simulink model "Rocket_Simulation"  (R2024a)
settings: Solver=VariableStepAuto  StartTime=0.0  StopTime=30  RelTol=1e-3
values from neighbouring files (symbols this model uses):
  g = -9.80665    [OpenRocketDataLoader.m]
libraries: simulink x1, aerolibactuator x1, aerolibatmos2 x1
settings Model: Creator=bennettbabu  LastModifiedBy=bennettbabu

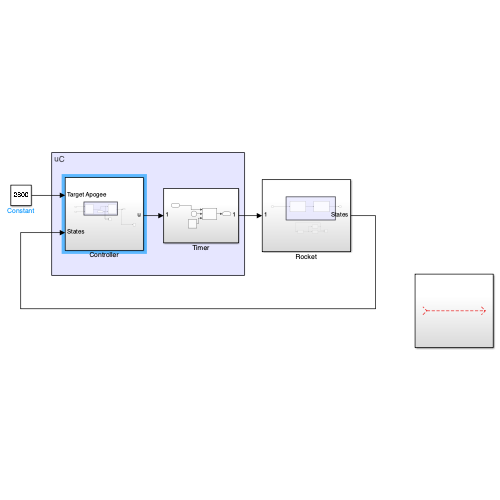
[thumbnail: Simulink's stored preview of the top-level diagram]
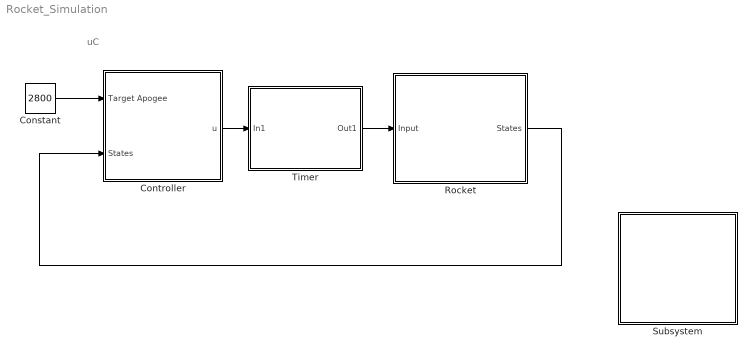
== system Rocket_Simulation ==
  note: uC
  Constant : Constant  Value=2800
  Controller : Subsystem
  Rocket : Subsystem
  Subsystem : Subsystem
  Timer : Subsystem
  wires:
  Rocket/1(States) -> Controller/2(States)
  Constant/1 -> Controller/1(Target Apogee)
  Controller/1(u) -> Timer/1(In1)
  Timer/1(Out1) -> Rocket/1(Input)

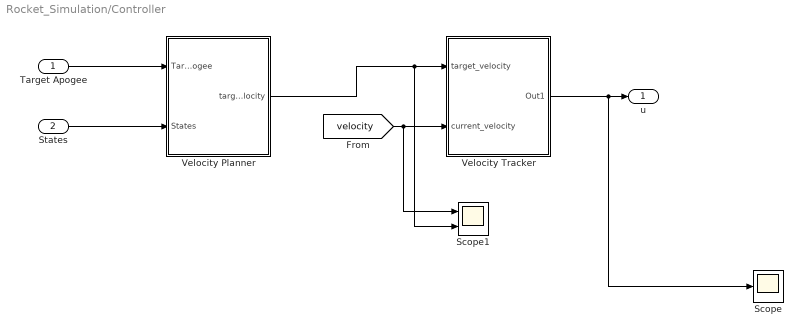
== system Rocket_Simulation/Controller ==
  Target Apogee : Inport
  States : Inport  Port=2
  Scope : Scope
  Scope1 : Scope  NumInputPorts=2
  Velocity Planner : Subsystem
  Velocity Tracker : Subsystem
  u : Outport
  wires:
  Target Apogee/1 -> Velocity Planner/1(Target Apogee)
  States/1 -> Velocity Planner/2(States)
  Velocity Tracker/1(Out1) -> Scope/1, u/1
  [velocity] -> Scope1/1, Velocity Tracker/2(current_velocity)
  Velocity Planner/1(target_velocity) -> Scope1/2, Velocity Tracker/1(target_velocity)

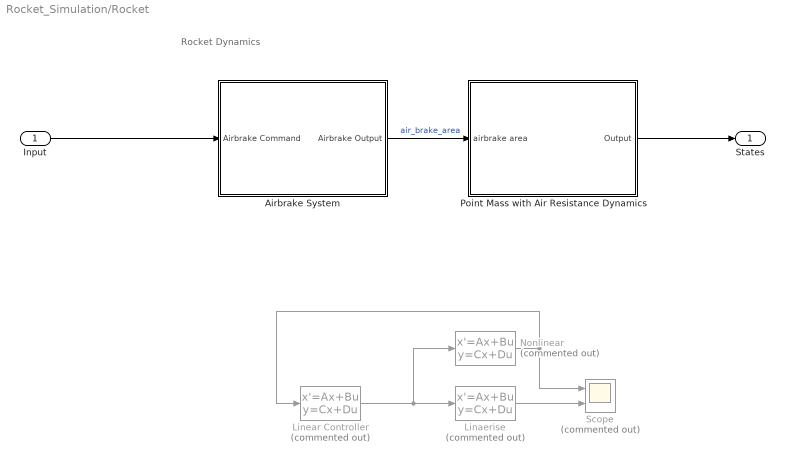
== system Rocket_Simulation/Rocket ==
  note: Rocket Dynamics
  Input : Inport
  Airbrake System : Subsystem
      mask Display: image('airbrake.png');
  "Linaerise " : StateSpace  Commented=on  InitialCondition=0
  Linear Controller : StateSpace  Commented=on  InitialCondition=0
  Nonlinear : StateSpace  Commented=on  InitialCondition=0
  "Point Mass with Air Resistance Dynamics " : Subsystem
      mask Display: image('rocket.jpeg');
  Scope : Scope  Commented=on  NumInputPorts=2
  States : Outport
  wires:
  "Point Mass with Air Resistance Dynamics "/1(Output) -> States/1
  Linear Controller/1 -> Nonlinear/1, "Linaerise "/1
  Nonlinear/1 -> Linear Controller/1, Scope/1
  "Linaerise "/1 -> Scope/2
  Input/1 -> Airbrake System/1(Airbrake Command)
  Airbrake System/1(Airbrake Output) -> "Point Mass with Air Resistance Dynamics "/1(airbrake area)  "air_brake_area"

== system Rocket_Simulation/Subsystem ==
  wires:
  ? -> ?

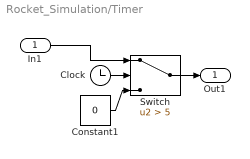
== system Rocket_Simulation/Timer ==
  In1 : Inport
  Clock : Clock
  Constant1 : Constant  Value=0
  Switch : Switch  Criteria=u2 > Threshold  Threshold=5  SaturateOnIntegerOverflow=off  InputSameDT=off
  Out1 : Outport
  wires:
  Switch/1 -> Out1/1
  Clock/1 -> Switch/2
  In1/1 -> Switch/1
  Constant1/1 -> Switch/3

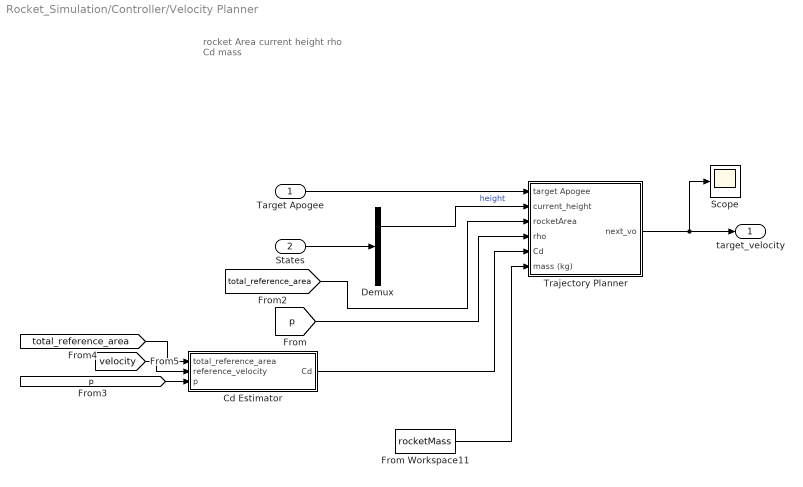
== system Rocket_Simulation/Controller/Velocity Planner ==
  note: rocket Area
      | current height
      | rho
      | Cd
      | mass
  Target Apogee : Inport
  States : Inport  Port=2
  Cd Estimator : Subsystem
  Demux : Demux  Outputs=2
  From Workspace11 : FromWorkspace  VariableName=rocketMass
  Scope : Scope
  Trajectory Planner : Subsystem
  target_velocity : Outport
  wires:
  States/1 -> Demux/1
  Demux/1 -> Trajectory Planner/2(current_height)  "height"
  Target Apogee/1 -> Trajectory Planner/1(target Apogee)
  [p] -> Trajectory Planner/4(rho)
  From Workspace11/1 -> Trajectory Planner/6(mass (kg))
  [p] -> Cd Estimator/3(p)
  [velocity] -> Cd Estimator/2(reference_velocity)
  [total_reference_area] -> Cd Estimator/1(total_reference_area)
  [total_reference_area] -> Trajectory Planner/3(rocketArea)
  Trajectory Planner/1(next_vo) -> Scope/1, target_velocity/1
  Cd Estimator/1(Cd) -> Trajectory Planner/5(Cd)

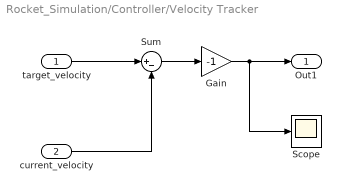
== system Rocket_Simulation/Controller/Velocity Tracker ==
  target_velocity : Inport
  current_velocity : Inport  Port=2
  Gain : Gain  Gain=-1
  Scope : Scope
  Sum : Sum  Inputs=|+-
  Out1 : Outport
  wires:
  Gain/1 -> Scope/1, Out1/1
  target_velocity/1 -> Sum/1
  current_velocity/1 -> Sum/2
  Sum/1 -> Gain/1

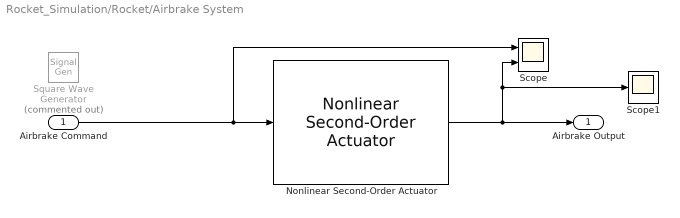
== system Rocket_Simulation/Rocket/Airbrake System ==
  Airbrake Command : Inport
  Nonlinear Second-Order Actuator : aerolibactuator/Nonlinear Second-Order Actuator  wn_fin=10  z_fin=0.7  fin_max=maxAirbrakeArea  fin_min=0  fin_maxrate=0.4  fin_act_0=0  fin_act_vel=0
  Scope : Scope  NumInputPorts=2
  Scope1 : Scope
  Square Wave Generator : SignalGenerator  Commented=on  WaveForm=square  Amplitude=0.01  Units=rad/sec
  Airbrake Output : Outport
  wires:
  Nonlinear Second-Order Actuator/1 -> Scope1/1, Scope/2, Airbrake Output/1
  Airbrake Command/1 -> Nonlinear Second-Order Actuator/1, Scope/1

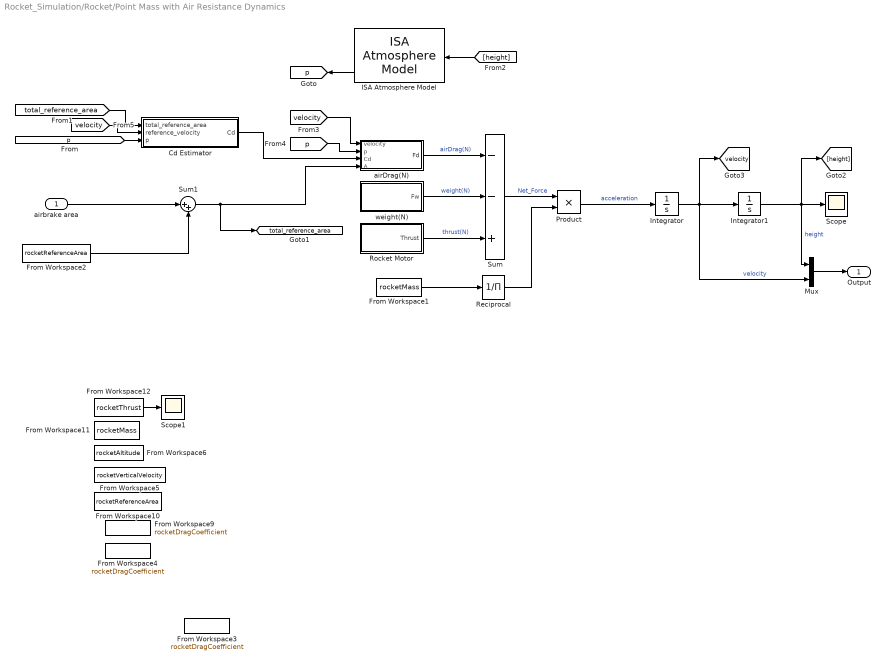
== system Rocket_Simulation/Rocket/Point Mass with Air Resistance Dynamics  ==
  airbrake area : Inport
  Cd Estimator : Subsystem
  From Workspace1 : FromWorkspace  VariableName=rocketMass
  From Workspace10 : FromWorkspace  VariableName=rocketReferenceArea
  From Workspace11 : FromWorkspace  VariableName=rocketMass
  From Workspace12 : FromWorkspace  VariableName=rocketThrust
  From Workspace2 : FromWorkspace  VariableName=rocketReferenceArea
  From Workspace3 : FromWorkspace  VariableName=rocketDragCoefficient
  From Workspace4 : FromWorkspace  VariableName=rocketDragCoefficient
  From Workspace5 : FromWorkspace  VariableName=rocketVerticalVelocity
  From Workspace6 : FromWorkspace  VariableName=rocketAltitude
  From Workspace9 : FromWorkspace  VariableName=rocketDragCoefficient
  ISA Atmosphere Model : aerolibatmos2/ISA Atmosphere Model  useExtended=off  action=Warning  custom=off  viscosityOut=off  g=9.80665  gamma=1.4  R=287.0531  L=0.0065  h_trop=11000  h_strat=20000  rho0=1.225  P0=101325  T0=288.15  h0=0  S=110.4  Tref=273.15  muref=1.716e-5
  Integrator : Integrator
  Integrator1 : Integrator
  Mux : Mux  Inputs=2
  Product : Product
  Reciprocal : Product  Inputs=/
  "Rocket Motor " : Subsystem
  Scope : Scope
  Scope1 : Scope
  Sum : Sum  Inputs=--+
  Sum1 : Sum  Inputs=|++
  airDrag(N) : Subsystem
  weight(N) : Subsystem
  Output : Outport
  tag scope: p=global, total_reference_area=global, velocity=global
  wires:
  "Rocket Motor "/1(Thrust) -> Sum/3  "thrust(N)"
  airDrag(N)/1(Fd) -> Sum/1  "airDrag(N)"
  weight(N)/1(Fw) -> Sum/2  "weight(N)"
  Sum/1 -> Product/1  "Net_Force"
  [p] -> Cd Estimator/3(p)
  ISA Atmosphere Model/4 -> [p]
  [total_reference_area] -> Cd Estimator/1(total_reference_area)
  [height] -> ISA Atmosphere Model/1
  [velocity] -> airDrag(N)/1(velocity)
  [p] -> airDrag(N)/2(p)
  Product/1 -> Integrator/1  "acceleration"
  Integrator/1 -> [velocity], Integrator1/1, Mux/2  "velocity"
  Integrator1/1 -> Mux/1, [height], Scope/1  "height"
  Mux/1 -> Output/1
  [velocity] -> Cd Estimator/2(reference_velocity)
  Reciprocal/1 -> Product/2
  From Workspace1/1 -> Reciprocal/1
  From Workspace12/1 -> Scope1/1
  airbrake area/1 -> Sum1/1
  Sum1/1 -> [total_reference_area], airDrag(N)/4(A)
  From Workspace2/1 -> Sum1/2
  Cd Estimator/1(Cd) -> airDrag(N)/3(Cd)

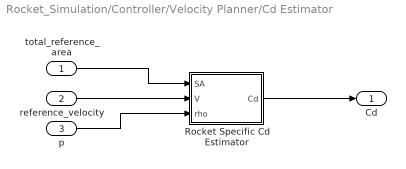
== system Rocket_Simulation/Controller/Velocity Planner/Cd Estimator ==
  total_reference_area : Inport
  reference_velocity : Inport  Port=2
  p : Inport  Port=3
  Rocket Specific Cd Estimator : MATLAB Function  TreatAsAtomicUnit=on
  Cd : Outport
  wires:
  Rocket Specific Cd Estimator/1(Cd) -> Cd/1
  total_reference_area/1 -> Rocket Specific Cd Estimator/1(SA)
  reference_velocity/1 -> Rocket Specific Cd Estimator/2(V)
  p/1 -> Rocket Specific Cd Estimator/3(rho)

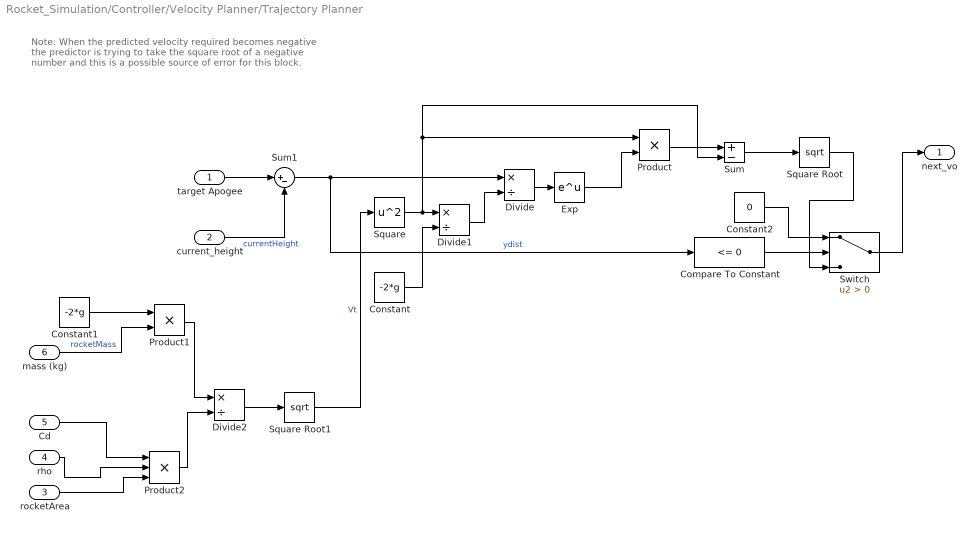
== system Rocket_Simulation/Controller/Velocity Planner/Trajectory Planner ==
  note: Note: When the predicted velocity required becomes negative the predictor is trying to take the square root of a negative number and this is a possible source of error for this block.
  target Apogee : Inport
  current_height : Inport  Port=2
  rocketArea : Inport  Port=3
  rho : Inport  Port=4
  Cd : Inport  Port=5
  mass (kg) : Inport  Port=6
  Compare To Constant : simulink/Logic and Bit Operations/Compare To Constant  relop=<=  const=0  OutDataTypeStr=boolean
  Constant : Constant  Value=-2*g
  Constant1 : Constant  Value=-2*g
  Constant2 : Constant  Value=0
  Divide : Product  Inputs=*/
  Divide1 : Product  Inputs=*/
  Divide2 : Product  Inputs=*/
  Exp : Math
  Product : Product
  Product1 : Product
  Product2 : Product  Inputs=3
  Square : Math  Operator=square
  Square Root : Sqrt
  Square Root1 : Sqrt
  Sum : Sum  Inputs=+-
  Sum1 : Sum  Inputs=|+-
  Switch : Switch  Criteria=u2 > Threshold  SaturateOnIntegerOverflow=off  InputSameDT=off
  next_vo : Outport
  wires:
  Sum/1 -> Square Root/1
  Product/1 -> Sum/1
  Exp/1 -> Product/2
  Divide/1 -> Exp/1
  Sum1/1 -> Compare To Constant/1, Divide/1  "ydist"
  Constant/1 -> Divide1/2
  Divide1/1 -> Divide/2
  Square/1 -> Sum/2, Product/1, Divide1/1
  target Apogee/1 -> Sum1/1
  Product2/1 -> Divide2/2
  Square Root1/1 -> Square/1  "Vt"
  Cd/1 -> Product2/1
  Divide2/1 -> Square Root1/1
  rocketArea/1 -> Product2/3
  Product1/1 -> Divide2/1
  Constant1/1 -> Product1/1
  rho/1 -> Product2/2
  mass (kg)/1 -> Product1/2  "rocketMass"
  current_height/1 -> Sum1/2  "currentHeight"
  Compare To Constant/1 -> Switch/2
  Constant2/1 -> Switch/1
  Square Root/1 -> Switch/3
  Switch/1 -> next_vo/1

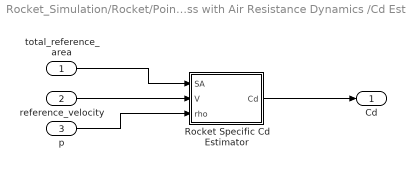
== system Rocket_Simulation/Rocket/Point Mass with Air Resistance Dynamics /Cd Estimator ==
  total_reference_area : Inport
  reference_velocity : Inport  Port=2
  p : Inport  Port=3
  Rocket Specific Cd Estimator : MATLAB Function  TreatAsAtomicUnit=on
  Cd : Outport
  wires:
  Rocket Specific Cd Estimator/1(Cd) -> Cd/1
  total_reference_area/1 -> Rocket Specific Cd Estimator/1(SA)
  reference_velocity/1 -> Rocket Specific Cd Estimator/2(V)
  p/1 -> Rocket Specific Cd Estimator/3(rho)

== system Rocket_Simulation/Rocket/Point Mass with Air Resistance Dynamics /Rocket Motor  ==
  From Workspace12 : FromWorkspace  VariableName=rocketThrust
  Thrust : Outport
  wires:
  From Workspace12/1 -> Thrust/1

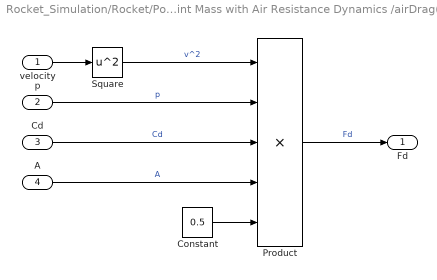
== system Rocket_Simulation/Rocket/Point Mass with Air Resistance Dynamics /airDrag(N) ==
  velocity : Inport
  p : Inport  Port=2
  Cd : Inport  Port=3
  A : Inport  Port=4
  Constant : Constant  Value=0.5
  Product : Product  Inputs=5
  Square : Math  Operator=square
  Fd : Outport
  wires:
  velocity/1 -> Square/1
  Square/1 -> Product/1  "v^2"
  p/1 -> Product/2  "p"
  Cd/1 -> Product/3  "Cd"
  A/1 -> Product/4  "A"
  Constant/1 -> Product/5
  Product/1 -> Fd/1  "Fd"

== system Rocket_Simulation/Rocket/Point Mass with Air Resistance Dynamics /weight(N) ==
  From Workspace11 : FromWorkspace  VariableName=rocketMass
  gravity : Gain  Gain=9.80665
  Fw : Outport
  wires:
  From Workspace11/1 -> gravity/1
  gravity/1 -> Fw/1

== matlab function Rocket_Simulation/Rocket/Point Mass with Air Resistance Dynamics /Cd Estimator/Rocket Specific Cd Estimator ==
  data: SA input; Cd output; V input; rho input
function Cd = fcn(SA,V,rho)
u1 =  43.32270126;  % Total rocket SA.
u2 = -0.000687709; % Velocity
u3 = 0.531869262; % Air density
intercept = -0.447146101;
Cd = (SA*u1)+ (V*u2)+ (rho*u3) + (intercept) ;
end

== matlab function Rocket_Simulation/Controller/Velocity Planner/Cd Estimator/Rocket Specific Cd Estimator ==
  data: SA input; Cd output; V input; rho input
function Cd = fcn(SA,V,rho)
u1 =  43.32270126;  % Total rocket SA.
u2 = -0.000687709; % Velocity
u3 = 0.531869262; % Air density
intercept = -0.447146101;
Cd = (SA*u1)+ (V*u2)+ (rho*u3) + (intercept) ;
end
